simulink library "util_integrator_lib"  (R2014b)
settings: Solver=ode45  SolverMode=SingleTasking  StartTime=0.0  StopTime=10.0  RelTol=1e-3
undefined symbols (not defined in the file): sim_time_step_size
libraries: util_integrator_lib x4, util_frame_rotation_lib x1, csu_grs_gravity_r_squared_lib x1
settings Model: Creator=hcannon  LastModifiedBy=mstewart

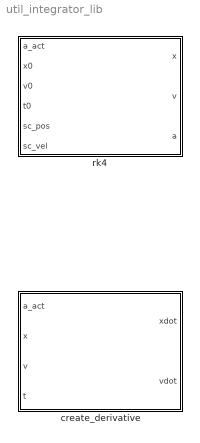
== system util_integrator_lib ==
  create_derivative : Subsystem
      mask Display:
      | disp('xdot(x)')
      | color('blue')
      | text(0.05,0.02,'MoonEx',...
      |  	'HorizontalAlignment','Left',...
      | 	'VerticalAlignment','bottom')
  rk4 : Subsystem  mask{DT=sim_time_step_size}
      mask prompts: DT "Time Step Size"
      mask Display:
      | disp('rk4(x)')
      | color('blue')
      | text(0.05,0.02,'MoonEx',...
      |  	'HorizontalAlignment','Left',...
      | 	'VerticalAlignment','bottom')

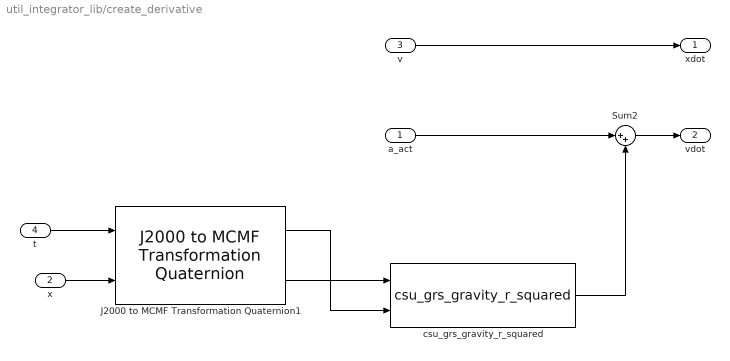
== system util_integrator_lib/create_derivative ==
  a_act : Inport
  x : Inport  Port=2
  v : Inport  Port=3
  t : Inport  Port=4
  J2000 to MCMF Transformation Quaternion1 : util_frame_rotation_lib/J2000 to MCMF  Transformation Quaternion  SystemSampleTime=-1
  Sum2 : Sum  Inputs=|++
  csu_grs_gravity_r_squared : csu_grs_gravity_r_squared_lib/csu_grs_gravity_r_squared  mu_central_body=central_body_gravity_mu
  xdot : Outport
  vdot : Outport  Port=2
  wires:
  v/1 -> xdot/1
  Sum2/1 -> vdot/1
  a_act/1 -> Sum2/1
  t/1 -> J2000 to MCMF Transformation Quaternion1/1
  x/1 -> J2000 to MCMF Transformation Quaternion1/2
  J2000 to MCMF Transformation Quaternion1/2 -> csu_grs_gravity_r_squared/1
  J2000 to MCMF Transformation Quaternion1/1 -> csu_grs_gravity_r_squared/2
  csu_grs_gravity_r_squared/1 -> Sum2/2

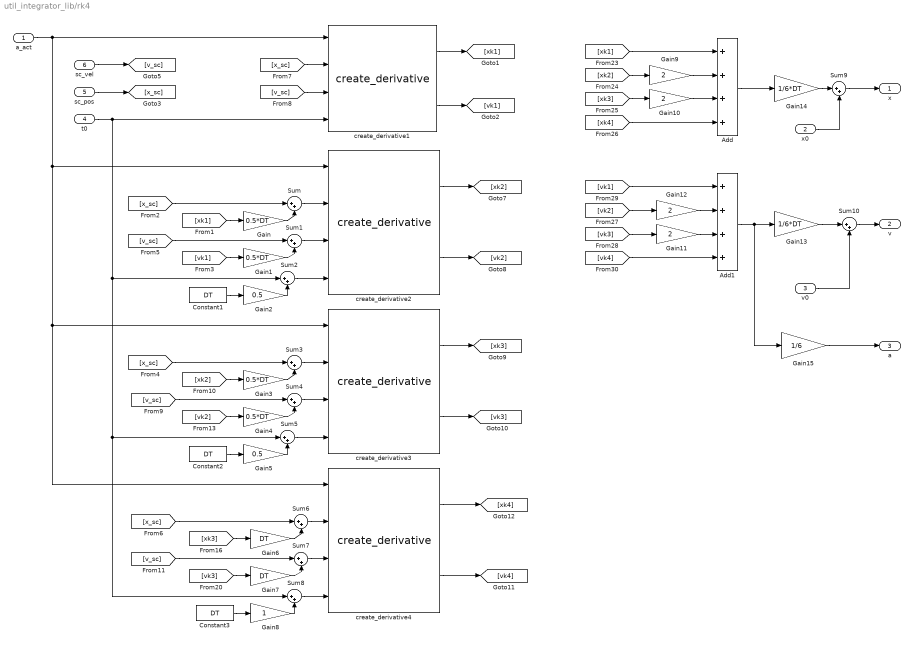
== system util_integrator_lib/rk4 ==
  a_act : Inport
  x0 : Inport  Port=2
  v0 : Inport  Port=3
  t0 : Inport  Port=4
  sc_pos : Inport  Port=5
  sc_vel : Inport  Port=6
  Add : Sum  Inputs=++++
  Add1 : Sum  Inputs=++++
  Constant1 : Constant  Value=DT
  Constant2 : Constant  Value=DT
  Constant3 : Constant  Value=DT
  Gain{,1,3..4} (4 alike) : Gain  Gain=0.5*DT
  Gain{9..12} (4 alike) : Gain  Gain=2
  Gain13 : Gain  Gain=1/6*DT
  Gain14 : Gain  Gain=1/6*DT
  Gain15 : Gain  Gain=1/6
  Gain2 : Gain  Gain=0.5
  Gain5 : Gain  Gain=0.5
  Gain6 : Gain  Gain=DT
  Gain7 : Gain  Gain=DT
  Gain8 : Gain
  Sum{,1..10} (11 alike) : Sum  Inputs=|++
  create_derivative{1..4} (4 alike) : util_integrator_lib/create_derivative  SystemSampleTime=-1
  x : Outport
  v : Outport  Port=2
  a : Outport  Port=3
  wires:
  [v_sc] -> Sum7/1
  [v_sc] -> Sum4/1
  [v_sc] -> Sum1/1
  [v_sc] -> create_derivative1/3
  sc_vel/1 -> [v_sc]
  sc_pos/1 -> [x_sc]
  create_derivative1/1 -> [xk1]
  create_derivative1/2 -> [vk1]
  Sum/1 -> create_derivative2/2
  [xk1] -> Gain/1
  [vk1] -> Gain1/1
  Gain/1 -> Sum/2
  Gain1/1 -> Sum1/2
  Sum1/1 -> create_derivative2/3
  [x_sc] -> Sum/1
  Sum2/1 -> create_derivative2/4
  Constant1/1 -> Gain2/1
  Gain2/1 -> Sum2/2
  [x_sc] -> create_derivative1/2
  t0/1 -> create_derivative1/4, Sum8/1, Sum5/1, Sum2/1
  create_derivative2/1 -> [xk2]
  create_derivative2/2 -> [vk2]
  Sum3/1 -> create_derivative3/2
  [xk2] -> Gain3/1
  [vk2] -> Gain4/1
  Gain3/1 -> Sum3/2
  Gain4/1 -> Sum4/2
  Sum4/1 -> create_derivative3/3
  [x_sc] -> Sum3/1
  Sum5/1 -> create_derivative3/4
  Constant2/1 -> Gain5/1
  Gain5/1 -> Sum5/2
  create_derivative3/1 -> [xk3]
  create_derivative3/2 -> [vk3]
  a_act/1 -> create_derivative1/1, create_derivative4/1, create_derivative3/1, create_derivative2/1
  Sum6/1 -> create_derivative4/2
  [xk3] -> Gain6/1
  [vk3] -> Gain7/1
  Gain6/1 -> Sum6/2
  Gain7/1 -> Sum7/2
  Sum7/1 -> create_derivative4/3
  [x_sc] -> Sum6/1
  Sum8/1 -> create_derivative4/4
  Constant3/1 -> Gain8/1
  Gain8/1 -> Sum8/2
  create_derivative4/1 -> [xk4]
  create_derivative4/2 -> [vk4]
  [xk2] -> Gain9/1
  [xk3] -> Gain10/1
  [xk1] -> Add/1
  Gain9/1 -> Add/2
  Gain10/1 -> Add/3
  [xk4] -> Add/4
  Gain12/1 -> Add1/2
  Gain11/1 -> Add1/3
  [vk4] -> Add1/4
  [vk2] -> Gain12/1
  [vk3] -> Gain11/1
  [vk1] -> Add1/1
  Add1/1 -> Gain15/1, Gain13/1
  Add/1 -> Gain14/1
  Gain14/1 -> Sum9/1
  x0/1 -> Sum9/2
  Sum9/1 -> x/1
  Gain13/1 -> Sum10/1
  Sum10/1 -> v/1
  v0/1 -> Sum10/2
  Gain15/1 -> a/1
